simulink model "oscillator3_ideal_2016a"  (R2016a)
settings: Solver=VariableStepAuto  SolverMode=SingleTasking  StartTime=0.0  StopTime=t_stop  RelTol=1e-3
values from neighbouring files (symbols this model uses):
  ts = 1/fs    (= 5.96046447754e-08)    [oscillator_sim.m]
  x0 = fs*[1;0]    [oscillator_sim.m]
settings Model: Creator=joseph  LastModifiedBy=rboon
settings DebuggingCC: SFUnexpectedBacktrackingDiag=error  SFNoUnconditionalDefaultTransitionDiag=error
settings SFSimCC: SimUseLocalCustomCode=on
settings RTWCC: RTWUseLocalCustomCode=on
settings GRTTargetCC: TargetLangStandard=C99 (ISO)  GeneratePreprocessorConditionals=Use local settings
settings ConfigComp: CovMetricSettings=dwe  CovHtmlReporting=off  CovSaveCumulativeToWorkspaceVar=off  CovSaveSingleToWorkspaceVar=off  CovExternalEMLEnable=on

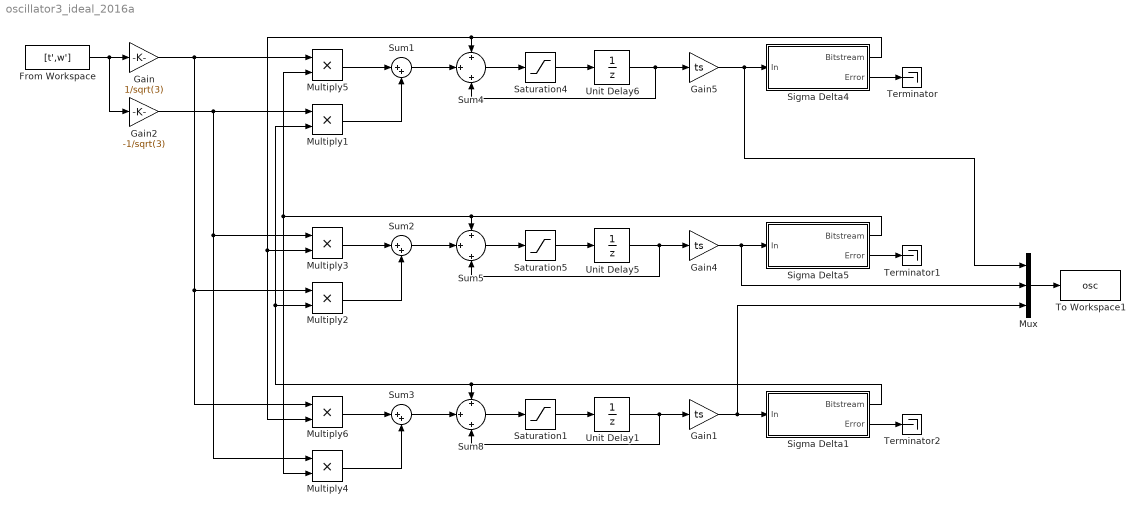
== system oscillator3_ideal_2016a ==
  From Workspace : FromWorkspace  VariableName=[t',w']  SampleTime=ts
  Gain : Gain  Gain=1/sqrt(3)
  Gain1 : Gain  Gain=ts
  Gain2 : Gain  Gain=-1/sqrt(3)
  Gain4 : Gain  Gain=ts
  Gain5 : Gain  Gain=ts
  Multiply{1..6} (6 alike) : Product
  Mux : Mux  Inputs=3
  Saturation1 : Saturate  UpperLimit=1/ts  LowerLimit=-1/ts
  Saturation4 : Saturate  UpperLimit=1/ts  LowerLimit=-1/ts
  Saturation5 : Saturate  UpperLimit=1/ts  LowerLimit=-1/ts
  Sigma Delta1 : Subsystem
  Sigma Delta4 : Subsystem
  Sigma Delta5 : Subsystem
  Sum1 : Sum  Inputs=|++
  Sum2 : Sum  Inputs=|++
  Sum3 : Sum  Inputs=|++
  Sum4 : Sum  Inputs=+|+|+
  Sum5 : Sum  Inputs=+|+|+
  Sum8 : Sum  Inputs=+|+|+
  Terminator : Terminator
  Terminator1 : Terminator
  Terminator2 : Terminator
  To Workspace1 : ToWorkspace  VariableName=osc  SampleTime=-1
      settings: Save2DSignal=2-D array (concatenate along first dimension)
  Unit Delay1 : UnitDelay  InitialCondition=x0(3)  SampleTime=ts  HasFrameUpgradeWarning=on
  Unit Delay5 : UnitDelay  InitialCondition=x0(2)  SampleTime=ts  HasFrameUpgradeWarning=on
  Unit Delay6 : UnitDelay  InitialCondition=x0(1)  SampleTime=ts  HasFrameUpgradeWarning=on
  wires:
  Gain5/1 -> Mux/1, Sigma Delta4/1(In)
  Sum4/1 -> Saturation4/1
  Unit Delay6/1 -> Sum4/3, Gain5/1
  Sum5/1 -> Saturation5/1
  Mux/1 -> To Workspace1/1
  Sigma Delta4/2(Error) -> Terminator/1
  Sigma Delta5/2(Error) -> Terminator1/1
  Sigma Delta1/2(Error) -> Terminator2/1
  Unit Delay5/1 -> Sum5/3, Gain4/1
  Unit Delay1/1 -> Sum8/3, Gain1/1
  Sum8/1 -> Saturation1/1
  Multiply5/1 -> Sum1/1
  Multiply1/1 -> Sum1/2
  Gain4/1 -> Mux/2, Sigma Delta5/1(In)
  Gain1/1 -> Mux/3, Sigma Delta1/1(In)
  Sum1/1 -> Sum4/2
  Sum2/1 -> Sum5/2
  Multiply2/1 -> Sum2/2
  Multiply3/1 -> Sum2/1
  Sum3/1 -> Sum8/2
  Multiply4/1 -> Sum3/2
  Multiply6/1 -> Sum3/1
  Gain/1 -> Multiply6/1, Multiply2/1, Multiply5/1
  Gain2/1 -> Multiply3/1, Multiply4/1, Multiply1/1
  Sigma Delta5/1(Bitstream) -> Multiply5/2, Multiply4/2, Sum5/1
  Sigma Delta1/1(Bitstream) -> Multiply2/2, Multiply1/2, Sum8/1
  Sigma Delta4/1(Bitstream) -> Multiply3/2, Multiply6/2, Sum4/1
  From Workspace/1 -> Gain2/1, Gain/1
  Saturation4/1 -> Unit Delay6/1
  Saturation5/1 -> Unit Delay5/1
  Saturation1/1 -> Unit Delay1/1

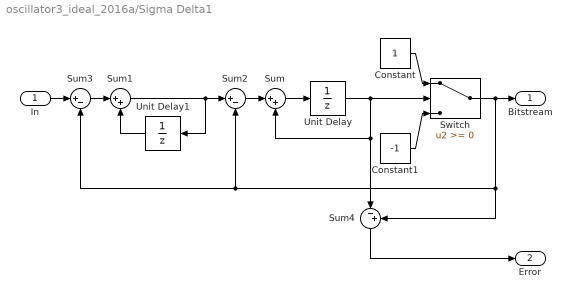
== system oscillator3_ideal_2016a/Sigma Delta1 ==
  In : Inport
  Constant : Constant
  Constant1 : Constant  Value=-1
  Sum : Sum  Inputs=|++
  Sum1 : Sum  Inputs=|++
  Sum2 : Sum  Inputs=|+-
  Sum3 : Sum  Inputs=|+-
  Sum4 : Sum  Inputs=|-+
  Switch : Switch
  Unit Delay : UnitDelay  SampleTime=ts  HasFrameUpgradeWarning=on
  Unit Delay1 : UnitDelay  SampleTime=ts  HasFrameUpgradeWarning=on
  Bitstream : Outport
  Error : Outport  Port=2
  wires:
  Sum4/1 -> Error/1
  Sum3/1 -> Sum1/1
  Constant1/1 -> Switch/3
  Unit Delay1/1 -> Sum1/2
  Sum/1 -> Unit Delay/1
  Unit Delay/1 -> Sum4/1, Sum/2, Switch/2
  Constant/1 -> Switch/1
  In/1 -> Sum3/1
  Sum2/1 -> Sum/1
  Sum1/1 -> Sum2/1, Unit Delay1/1
  Switch/1 -> Sum4/2, Sum3/2, Sum2/2, Bitstream/1

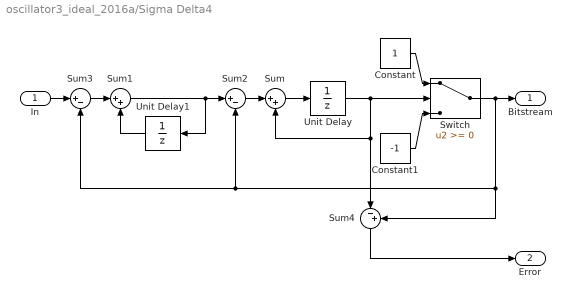
== system oscillator3_ideal_2016a/Sigma Delta4 ==
  In : Inport
  Constant : Constant
  Constant1 : Constant  Value=-1
  Sum : Sum  Inputs=|++
  Sum1 : Sum  Inputs=|++
  Sum2 : Sum  Inputs=|+-
  Sum3 : Sum  Inputs=|+-
  Sum4 : Sum  Inputs=|-+
  Switch : Switch
  Unit Delay : UnitDelay  SampleTime=ts  HasFrameUpgradeWarning=on
  Unit Delay1 : UnitDelay  SampleTime=ts  HasFrameUpgradeWarning=on
  Bitstream : Outport
  Error : Outport  Port=2
  wires:
  Sum4/1 -> Error/1
  Sum3/1 -> Sum1/1
  Constant1/1 -> Switch/3
  Unit Delay1/1 -> Sum1/2
  Sum/1 -> Unit Delay/1
  Unit Delay/1 -> Sum4/1, Sum/2, Switch/2
  Constant/1 -> Switch/1
  In/1 -> Sum3/1
  Sum2/1 -> Sum/1
  Sum1/1 -> Sum2/1, Unit Delay1/1
  Switch/1 -> Sum4/2, Sum3/2, Sum2/2, Bitstream/1

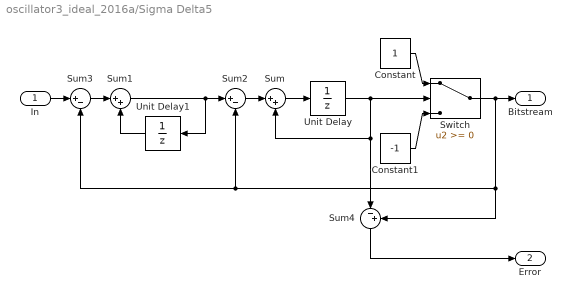
== system oscillator3_ideal_2016a/Sigma Delta5 ==
  In : Inport
  Constant : Constant
  Constant1 : Constant  Value=-1
  Sum : Sum  Inputs=|++
  Sum1 : Sum  Inputs=|++
  Sum2 : Sum  Inputs=|+-
  Sum3 : Sum  Inputs=|+-
  Sum4 : Sum  Inputs=|-+
  Switch : Switch
  Unit Delay : UnitDelay  SampleTime=ts  HasFrameUpgradeWarning=on
  Unit Delay1 : UnitDelay  SampleTime=ts  HasFrameUpgradeWarning=on
  Bitstream : Outport
  Error : Outport  Port=2
  wires:
  Sum4/1 -> Error/1
  Sum3/1 -> Sum1/1
  Constant1/1 -> Switch/3
  Unit Delay1/1 -> Sum1/2
  Sum/1 -> Unit Delay/1
  Unit Delay/1 -> Sum4/1, Sum/2, Switch/2
  Constant/1 -> Switch/1
  In/1 -> Sum3/1
  Sum2/1 -> Sum/1
  Sum1/1 -> Sum2/1, Unit Delay1/1
  Switch/1 -> Sum4/2, Sum3/2, Sum2/2, Bitstream/1
